simulink model "min_order_observer"  (R2025a)
settings: Solver=VariableStepAuto  StartTime=0.0  StopTime=10.0  RelTol=1e-3
values from neighbouring files (symbols this model uses):
  A_hat = A_bb - Ke*A_ab    [Controller.m]    (also in min_state_observer.m)
  B = [0 1/M 0 1/(M*l)]'    [CartPuller.m]    (also in Controller.m = [0;1/m1;0;0]; Ex12_4.m = [0;0;1]; Observer_4state.m = [0; 1/m]; full_order_observer_smd.m = [0 0 0 1/m2]')
  B_hat = A_hat*Ke + A_ba - Ke*A_aa    [Controller.m]    (also in min_state_observer.m)
  C = eye(4)    [Controller.m]    (also in Ex12_4.m = [-1 1 0]; Observer_4state.m = [1 0]; full_order_observer_smd.m = [1 0 0 0]; full_state_observer.m = [1 0 0 0])
  C_hat = [zeros(1, 3) ... (first row only)    [Controller.m]    (also in min_state_observer.m)
  D_hat = [1 ... (first row only)    [Controller.m]    (also in min_state_observer.m)
  F_hat = B_b - Ke*B_a    [Controller.m]    (also in min_state_observer.m)
  K = lqr(A,B,Q,R)    [CartPuller.m]    (also in Ex12_4.m = acker(A,B,poles); full_state_observer.m = place(A', C', poles_o)'; me23b196_asgn4.m = product_of_pole_magnitudes / product_of_zero_magnitudes)
settings Model: Creator=abhi  LastModifiedBy=abhi

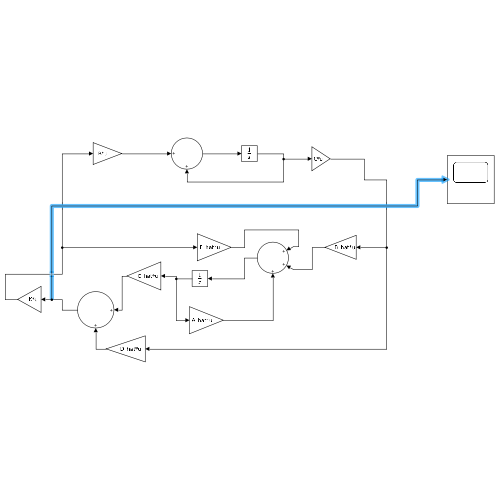
[thumbnail: Simulink's stored preview of the top-level diagram]
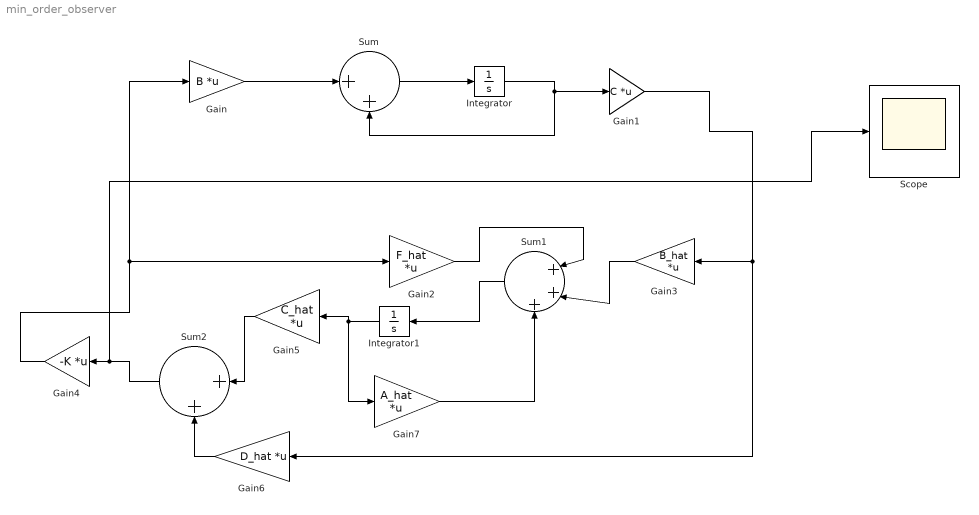
== system min_order_observer ==
  Gain : Gain  Gain=B  Multiplication=Matrix(K*u)
  Gain1 : Gain  Gain=C  Multiplication=Matrix(K*u)
  Gain2 : Gain  Gain=F_hat  Multiplication=Matrix(K*u)
  Gain3 : Gain  Gain=B_hat  Multiplication=Matrix(K*u)
  Gain4 : Gain  Gain=-K  Multiplication=Matrix(K*u)
  Gain5 : Gain  Gain=C_hat  Multiplication=Matrix(K*u)
  Gain6 : Gain  Gain=D_hat  Multiplication=Matrix(K*u)
  Gain7 : Gain  Gain=A_hat  Multiplication=Matrix(K*u)
  Integrator : Integrator
  Integrator1 : Integrator
  Scope : Scope
      settings: SampleTime=1e-5  ActiveDisplayYMinimum=-0.25738390800345695  ActiveDisplayYMaximum=0.317662888448862
  Sum : Sum  Inputs=|++
  Sum1 : Sum  Inputs=|+++
  Sum2 : Sum  Inputs=|++
  wires:
  Gain4/1 -> Gain/1, Gain2/1
  Gain/1 -> Sum/1
  Sum/1 -> Integrator/1
  Integrator/1 -> Sum/2, Gain1/1
  Gain1/1 -> Gain6/1, Gain3/1
  Gain3/1 -> Sum1/2
  Gain2/1 -> Sum1/1
  Gain6/1 -> Sum2/2
  Gain5/1 -> Sum2/1
  Sum2/1 -> Scope/1, Gain4/1
  Integrator1/1 -> Gain7/1, Gain5/1
  Gain7/1 -> Sum1/3
  Sum1/1 -> Integrator1/1
